simulink model "SolarTrackingModel"  (R2021b)
settings: Solver=ode4  StartTime=0.0  StopTime=50  RelTol=1e-3
settings Model: Creator=ASUS  LastModifiedBy=Shahbazi
settings OptimizationCC: DefaultParameterBehavior=Inlined  EnhancedBackFolding=on  PassReuseOutputArgsAs=Individual arguments  ZeroExternalMemoryAtStartup=off  ZeroInternalMemoryAtStartup=off  OptimizeBlockOrder=speed  DifferentSizesBufferReuse=on  OptimizationCustomize=off  EfficientTunableParamExpr=on
settings DebuggingCC: ParameterTunabilityLossMsg=error
settings SFSimCC: MATLABDynamicMemAlloc=off
settings RTWCC: Description=Embedded Coder  SystemTargetFile=ert.tlc  TemplateMakefile=ert_default_tmf  GenerateReport=on  LaunchReport=on
settings CodeAppCC: ForceParamTrailComments=on  IgnoreCustomStorageClasses=off  OperatorAnnotations=on  SimulinkDataObjDesc=on  SFDataObjDesc=on  InsertBlockDesc=on
settings ERTTargetCC: TargetLangStandard=C99 (ISO)  GenerateSampleERTMain=on  InlinedParameterPlacement=NonHierarchical  ERTCustomFileTemplate=example_file_process.tlc

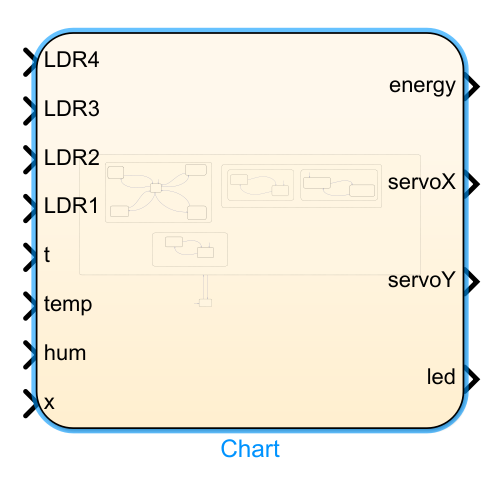
[thumbnail: Simulink's stored preview of the top-level diagram]
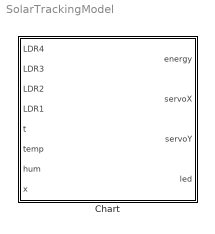
== system SolarTrackingModel ==
  Chart : Stateflow chart  TreatAsAtomicUnit=on

== stateflow chart SolarTrackingModel/Chart ==
  state PowerOn [parallel]
    settings: executionOrder=1
    state SunTracking [parallel]
      settings: executionOrder=1
      state MoveRight
        servoX = servoX + 1;
      state MoveLeft
        servoX = servoX - 1;
      state Idle
      state MoveUp
        servoY = servoY +1;
      state MoveDown
        servoY = servoY -1;
      MoveRight -> Idle : [(LDR2+LDR4) <= (LDR1+LDR3)]
      MoveLeft -> Idle : [(LDR1+LDR3) <= (LDR2+LDR4)]
      Idle -> MoveRight [order 1] : [(LDR2+LDR4) > (LDR1+LDR3)]
      Idle -> MoveLeft [order 2] : [(LDR1+LDR3) > (LDR2+LDR4)]
      (default) -> Idle
      MoveDown -> Idle : [(LDR3+LDR4) <= (LDR1+LDR2)]
      MoveUp -> Idle : [(LDR1+LDR2) <= (LDR3+LDR4)]
      Idle -> MoveUp [order 3] : [(LDR1+LDR2) > (LDR3+LDR4)]
      Idle -> MoveDown [order 4] : [(LDR3+LDR4) > (LDR1+LDR2)]
    state EnergyManagement [parallel]
      settings: executionOrder=2
      state EnergyLevel [parallel]
        settings: executionOrder=2
        state LowEnergy
          led = 1;
        state Normal
          led = 0;
        LowEnergy -> Normal : [energy >=20]
        (default) -> Normal
        Normal -> LowEnergy : [energy < 20]
      state DailyCycle [parallel]
        settings: executionOrder=1
        state Day
          energy = min(energy + 2, 100);
        state Night
          energy = max(energy / 1.3, 0);
        (default) -> Day
        Day -> Night : [t < 0]
        Night -> Day : [t >= 0]
    state EnvMonitoring [parallel]
      settings: executionOrder=3
      state Danger
        servoX = 90;
        servoY = 90;
      state Safe
      Danger -> Safe : [(temp <= 40 && hum <= 80)]
      (default) -> Safe
      Safe -> Danger : [(temp > 40 || hum > 80)]
  state PowerOff [parallel]
    settings: executionOrder=2
  PowerOff -> PowerOn : [x==1]
  PowerOn -> PowerOff : [x==0]
  (default) -> PowerOff
  data: LDR4 input; LDR3 input; LDR2 input; energy output =1; servoX output =90; LDR1 input; t input; servoY output =90; led output =0; temp input; hum input; x input
